simulink model "SimulinkModelGeneral_BAv03"  (R2023a)
settings: Solver=VariableStepAuto  StartTime=0.0  StopTime=1*3600  MaxStep=0.2  RelTol=1e-3
settings Model: NumberOfSteps=100  Creator=giaco  LastModifiedBy=giaco
settings OptimizationCC: ReuseModelBlockBuffer=off

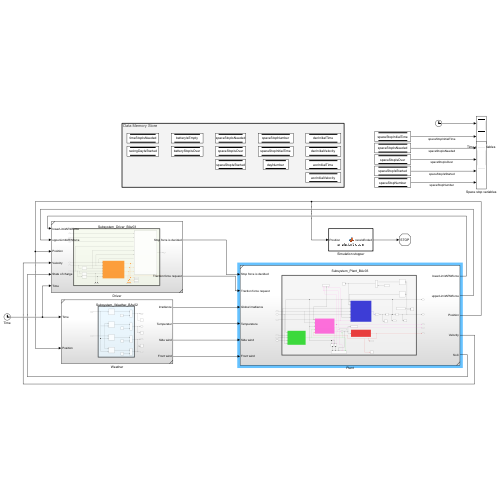
[thumbnail: Simulink's stored preview of the top-level diagram]
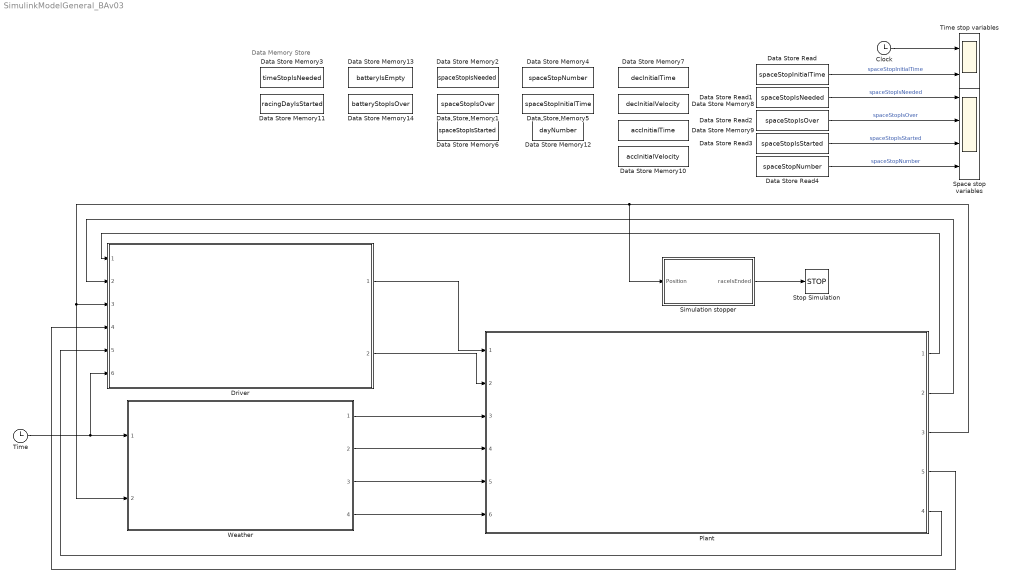
== system SimulinkModelGeneral_BAv03 ==
  note: Data Memory Store
  Clock : Clock
  Data Store Memory1 : DataStoreMemory  DataStoreName=spaceStopIsOver  WriteAfterWriteMsg=warning  InitialValue=false  ShowAdditionalParam=off  OutDataTypeStr=boolean
  Data Store Memory10 : DataStoreMemory  DataStoreName=accInitialVelocity  WriteAfterWriteMsg=warning  VectorParams1D=off  ShowAdditionalParam=off  OutDataTypeStr=double
  Data Store Memory11 : DataStoreMemory  DataStoreName=racingDayIsStarted  WriteAfterWriteMsg=warning  InitialValue=true  ShowAdditionalParam=off  OutDataTypeStr=boolean
  Data Store Memory12 : DataStoreMemory  DataStoreName=dayNumber  WriteAfterWriteMsg=warning  InitialValue=1  VectorParams1D=off  ShowAdditionalParam=off  OutDataTypeStr=double
  Data Store Memory13 : DataStoreMemory  DataStoreName=batteryIsEmpty  WriteAfterWriteMsg=warning  InitialValue=false  ShowAdditionalParam=off  OutDataTypeStr=boolean
  Data Store Memory14 : DataStoreMemory  DataStoreName=batteryStopIsOver  WriteAfterWriteMsg=warning  InitialValue=false  ShowAdditionalParam=off  OutDataTypeStr=boolean
  Data Store Memory2 : DataStoreMemory  DataStoreName=spaceStopIsNeeded  WriteAfterWriteMsg=warning  InitialValue=false  ShowAdditionalParam=off  OutDataTypeStr=boolean
  Data Store Memory3 : DataStoreMemory  DataStoreName=timeStopIsNeeded  WriteAfterWriteMsg=warning  InitialValue=false  ShowAdditionalParam=off  OutDataTypeStr=boolean
  Data Store Memory4 : DataStoreMemory  DataStoreName=spaceStopNumber  WriteAfterWriteMsg=warning  InitialValue=2  VectorParams1D=off  ShowAdditionalParam=off  OutDataTypeStr=double
  Data Store Memory5 : DataStoreMemory  DataStoreName=spaceStopInitialTime  WriteAfterWriteMsg=warning  VectorParams1D=off  ShowAdditionalParam=off  OutDataTypeStr=double
  Data Store Memory6 : DataStoreMemory  DataStoreName=spaceStopIsStarted  WriteAfterWriteMsg=warning  InitialValue=false  ShowAdditionalParam=off  OutDataTypeStr=boolean
  Data Store Memory7 : DataStoreMemory  DataStoreName=decInitialTime  WriteAfterWriteMsg=warning  VectorParams1D=off  ShowAdditionalParam=off  OutDataTypeStr=double
  Data Store Memory8 : DataStoreMemory  DataStoreName=decInitialVelocity  WriteAfterWriteMsg=warning  VectorParams1D=off  ShowAdditionalParam=off  OutDataTypeStr=double
  Data Store Memory9 : DataStoreMemory  DataStoreName=accInitialTime  WriteAfterWriteMsg=warning  VectorParams1D=off  ShowAdditionalParam=off  OutDataTypeStr=double
  Data Store Read : DataStoreRead  DataStoreName=spaceStopInitialTime  IndexOptions=Index vector (dialog)  Indices=1  OutputSizes=1
  Data Store Read1 : DataStoreRead  DataStoreName=spaceStopIsNeeded  IndexOptions=Index vector (dialog)  Indices=1  OutputSizes=1
  Data Store Read2 : DataStoreRead  DataStoreName=spaceStopIsOver  IndexOptions=Index vector (dialog)  Indices=1  OutputSizes=1
  Data Store Read3 : DataStoreRead  DataStoreName=spaceStopIsStarted  IndexOptions=Index vector (dialog)  Indices=1  OutputSizes=1
  Data Store Read4 : DataStoreRead  DataStoreName=spaceStopNumber  IndexOptions=Index vector (dialog)  Indices=1  OutputSizes=1
  Driver : Subsystem  ReferencedSubsystem=Subsystem_Driver_BAv03
  Plant : Subsystem  ReferencedSubsystem=Subsystem_Plant_BAv03
      settings: PortSchema="{\"entries\":[{\"content\":{\"sides\":[{\"content\":{\"connectorIds\":[\"In1\",\"In2\",\"In3\",\"In4\",\"In5\",\"In6\"]},\"type\":\"ConnectorPlacement.EquallySpacedRectSide\",\"uuid\":\"252d5260-9587-45a6-80e0-6a9716ce41a8\"},{\"content\":{\"connectorIds\":[\"Out1\",\"Out2\",\"Out3\",\"Out5\",\"Out4\"],\"side\":\"RIGHT\"},\"type\":\"ConnectorPlacement.EquallySpacedRectSide\",\"uuid\":\"3f90c69b-5a04-4e16-807d-5695fdf7e0ba\"},{\"content\":{\"side\":\"TOP\"},\"type\":\"ConnectorPlacement.EquallySpacedRectSide\",\"uuid\":\"0551eed8-5e0a-4ac1-9cbf-7bf8b5f56ba9\"}]},\"type\":\"ConnectorPlacement.EquallySpacedConnector\",\"uuid\":\"b830746a-2cd3-43fc-b647-58e1203a3694\"}],\"packageUris\":[\"http://schema.mathworks.com/mf0/Connector/R2020b\"],\"version\":\"1.0\"}"
  Simulation stopper : MATLAB Function  TreatAsAtomicUnit=on
  Space stop variables : Scope  NumInputPorts=4
  Stop Simulation : Stop
  Time : Clock
  Time stop variables : Scope  NumInputPorts=2
  Weather : Subsystem  ReferencedSubsystem=Subsystem_Weather_BAv02
  wires:
  Driver/2 -> Plant/2
  Weather/1 -> Plant/3
  Weather/2 -> Plant/4
  Weather/3 -> Plant/5
  Time/1 -> Driver/6, Weather/1
  Driver/1 -> Plant/1
  Plant/1 -> Driver/1
  Plant/2 -> Driver/2
  Plant/5 -> Driver/4
  Plant/4 -> Driver/5
  Weather/4 -> Plant/6
  Data Store Read/1 -> Time stop variables/2  "spaceStopInitialTime"
  Data Store Read2/1 -> Space stop variables/2  "spaceStopIsOver"
  Data Store Read3/1 -> Space stop variables/3  "spaceStopIsStarted"
  Data Store Read1/1 -> Space stop variables/1  "spaceStopIsNeeded"
  Data Store Read4/1 -> Space stop variables/4  "spaceStopNumber"
  Clock/1 -> Time stop variables/1
  Simulation stopper/1(raceIsEnded) -> Stop Simulation/1
  Plant/3 -> Simulation stopper/1(Position), Driver/3, Weather/2

== matlab function SimulinkModelGeneral_BAv03/Simulation stopper ==
  data: Position input; raceIsEnded output; driver parameter
function raceIsEnded = simulationStopper(Position, driver)

raceIsEnded = false;

if Position >= driver.finishLocDist
    raceIsEnded = true;
end % if
